simulink model "FDL_Trajectary_Tracking_SBR"  (R2021a)
settings: Solver=VariableStepAuto  StartTime=0.0  StopTime=50  FixedStep=0.01  RelTol=1e-6
values from neighbouring files (symbols this model uses):
  A_v = linear_SBR6voltage_A(I_W_a,I_y,R_m,g,k_e,k_m,l,m_B,m_W,r)    [lqr_control_3DOF.m]
  B_v = linear_SBR6voltage_B(I_W_a,I_W_d,I_y,I_z,R_m,d,k_m,l,m_B,m_W,r)    [lqr_control_3DOF.m]
  C = eye(6)    [lqr_control_3DOF.m]
  C_L = 0    [lqr_control_3DOF.m]
  d = 0.23    [lqr_control_3DOF.m]
  D = zeros(6,2)    [lqr_control_3DOF.m]
  g = 9.81    [lqr_control_3DOF.m]
  I_W_a = 0.0000365    (= 3.65e-05)    [lqr_control_3DOF.m]
  I_W_d = 0.00001825    (= 1.825e-05)    [lqr_control_3DOF.m]
  I_x = 0.007402    [lqr_control_3DOF.m]
  I_y = 0.00429462    [lqr_control_3DOF.m]
  I_z = 0.003350    (= 0.00335)    [lqr_control_3DOF.m]
  k_e = 0.63    [lqr_control_3DOF.m]
  k_m = 0.63    [lqr_control_3DOF.m]
  K_v = lqr(A_v,B_v,Q,R)    [lqr_control_3DOF.m]
  l = 0.045    [lqr_control_3DOF.m]
  m_B = 1.15    [lqr_control_3DOF.m]
  m_W = 0.053    [lqr_control_3DOF.m]
  r = 0.0425    [lqr_control_3DOF.m]
  R_m = 1.25    [lqr_control_3DOF.m]
libraries: aerolibutil x6, vrlib x1
settings Model: SimulationMode=accelerator  Creator=om  LastModifiedBy=jitt7
settings SolverCC: ConcurrentTasks=on  PositivePriorityOrder=on
settings DataIOCC: ReturnWorkspaceOutputs=off
settings OptimizationCC: BlockReduction=off  OptimizeBlockIOStorage=off
settings DebuggingCC: AlgebraicLoopMsg=none  ArtificialAlgebraicLoopMsg=none  SFMachineParentedDataDiag=warning  ArithmeticOperatorsInVariantConditions=warning
settings HardwareCC: ProdBitPerLong=64  ProdLongLongMode=on  ProdHWDeviceType=Intel->x86-64 (Linux 64)
settings SFSimCC: SimUseLocalCustomCode=off  CustomCodeUndefinedFunction=UseInterfaceOnly
settings RTWCC: Description=Simulink Real-Time  SystemTargetFile=slrealtime.tlc  TemplateMakefile=slrealtime_default_tmf  RTWUseLocalCustomCode=off  Toolchain=Simulink Real-Time Toolchain  BuildConfiguration=Faster Runs  CodeExecutionProfiling=on  TargetLang=C++

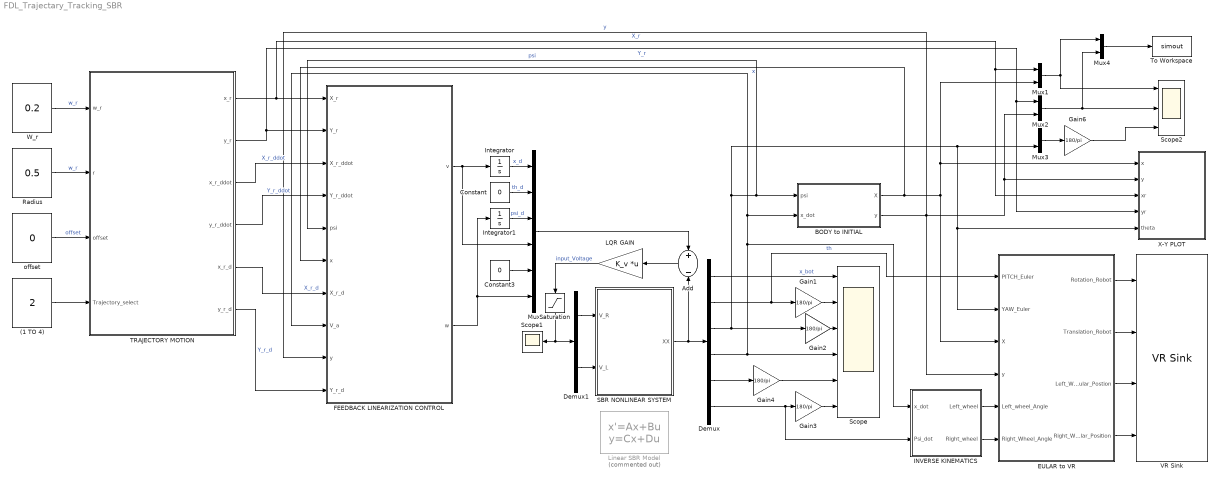
== system FDL_Trajectary_Tracking_SBR ==
  (1 TO 4) : Constant  Value=2
  Add : Sum  Inputs=+-
  BODY to INITIAL : Subsystem
  Constant : Constant  Value=0
  Constant3 : Constant  Value=0
  Demux : Demux  Outputs=6
  Demux1 : Demux  Outputs=2
  EULAR to VR : Subsystem
  FEEDBACK LINEARIZATION CONTROL : Subsystem
  Gain{1..4,6} (5 alike) : Gain  Gain=180/pi
  INVERSE KINEMATICS : Subsystem
  Integrator : Integrator
  Integrator1 : Integrator
  LQR GAIN : Gain  Gain=K_v  Multiplication=Matrix(K*u)
  Linear SBR Model : StateSpace  Commented=on  A=A_v  B=B_v  C=C  D=D  InitialCondition="[0  0  0  0 0 0]"
  Mux : Mux  Inputs=6
  Mux{1..4} (4 alike) : Mux  Inputs=2
  Radius : Constant  Value=0.5
  SBR NONLINEAR SYSTEM : Subsystem
  Saturation : Saturate  UpperLimit=12  LowerLimit=-12
  Scope : Scope  NumInputPorts=6
  Scope1 : Scope
  Scope2 : Scope  NumInputPorts=3
  TRAJECTORY MOTION : Subsystem
  To Workspace : ToWorkspace  VariableName=simout  SampleTime=-1
  VR Sink : vrlib/VR Sink  InstantiateOnLoad=on  SampleTime=0.05  ViewEnable=on  RemoteChange=off  RemoteView=off  FieldsWritten=__1.rotation.4.1.1.double#__1.translation.3.1.1.double#wheel-3.rotation.4.1.1.double#wheel-4.rotation.4.1.1.double  WorldFileName=JitendersirSBR.wrl  AutoView=off  VideoDimensions=[]  AllowVariableSize=off
  W_r : Constant  Value=0.2
  X-Y PLOT : MATLAB Function  TreatAsAtomicUnit=on
  offset : Constant  Value=0
  wires:
  Demux/6 -> INVERSE KINEMATICS/2(Psi_dot), Gain3/1
  Add/1 -> LQR GAIN/1
  Constant/1 -> Mux/2  "th_d"
  Demux/4 -> Scope/4, BODY to INITIAL/2(x_dot), FEEDBACK LINEARIZATION CONTROL/8(V_a), INVERSE KINEMATICS/1(x_dot)
  LQR GAIN/1 -> Saturation/1  "input_Voltage"
  Constant3/1 -> Mux/5
  Demux/2 -> EULAR to VR/1(PITCH_Euler), Gain1/1  "th"
  Demux/1 -> Scope/1  "x_bot"
  Mux/1 -> Add/1
  Gain4/1 -> Scope/5
  Demux/5 -> Gain4/1
  Gain1/1 -> Scope/2
  Gain2/1 -> Scope/3
  Integrator/1 -> Mux/1  "x_d"
  EULAR to VR/2(Translation_Robot) -> VR Sink/2
  EULAR to VR/4(Right_Wheel_Angular_Position) -> VR Sink/4
  EULAR to VR/3(Left_Wheel_Angular_Postion) -> VR Sink/3
  EULAR to VR/1(Rotation_Robot) -> VR Sink/1
  Mux1/1 -> Scope2/1, Mux4/1
  Mux2/1 -> Scope2/2, Mux4/2
  Mux3/1 -> Gain6/1
  Gain6/1 -> Scope2/3
  Demux1/1 -> SBR NONLINEAR SYSTEM/1(V_R)
  Demux1/2 -> SBR NONLINEAR SYSTEM/2(V_L)
  SBR NONLINEAR SYSTEM/1(XX) -> Demux/1, Add/2
  INVERSE KINEMATICS/1(Left_wheel) -> EULAR to VR/5(Left_wheel_Angle)
  INVERSE KINEMATICS/2(Right_wheel) -> EULAR to VR/6(Right_Wheel_Angle)
  BODY to INITIAL/1(X) -> FEEDBACK LINEARIZATION CONTROL/6(x), Mux1/2, X-Y PLOT/1(x), EULAR to VR/3(X)  "x"
  Mux4/1 -> To Workspace/1
  Saturation/1 -> Scope1/1, Demux1/1
  W_r/1 -> TRAJECTORY MOTION/1(w_r)  "w_r"
  TRAJECTORY MOTION/1(x_r) -> Mux1/1, X-Y PLOT/3(xr), FEEDBACK LINEARIZATION CONTROL/1(X_r)  "X_r"
  TRAJECTORY MOTION/2(y_r) -> Mux2/1, X-Y PLOT/4(yr), FEEDBACK LINEARIZATION CONTROL/2(Y_r)  "Y_r"
  BODY to INITIAL/2(y) -> FEEDBACK LINEARIZATION CONTROL/9(y), X-Y PLOT/2(y), Mux2/2, EULAR to VR/4(y)  "y"
  FEEDBACK LINEARIZATION CONTROL/1(v) -> Integrator/1, Mux/4
  FEEDBACK LINEARIZATION CONTROL/2(w) -> Integrator1/1, Mux/6
  TRAJECTORY MOTION/3(x_r_ddot) -> FEEDBACK LINEARIZATION CONTROL/3(X_r_ddot)  "X_r_ddot"
  TRAJECTORY MOTION/4(y_r_ddot) -> FEEDBACK LINEARIZATION CONTROL/4(Y_r_ddot)  "Y_r_ddot"
  TRAJECTORY MOTION/5(x_r_d) -> FEEDBACK LINEARIZATION CONTROL/7(X_r_d)  "X_r_d"
  TRAJECTORY MOTION/6(y_r_d) -> FEEDBACK LINEARIZATION CONTROL/10(Y_r_d)  "Y_r_d"
  offset/1 -> TRAJECTORY MOTION/3(offset)  "offset"
  Radius/1 -> TRAJECTORY MOTION/2(r)  "w_r"
  Demux/3 -> Gain2/1, BODY to INITIAL/1(psi), FEEDBACK LINEARIZATION CONTROL/5(psi), Mux3/2, EULAR to VR/2(YAW_Euler), X-Y PLOT/5(theta)  "psi"
  Integrator1/1 -> Mux/3  "psi_d"
  (1 TO 4)/1 -> TRAJECTORY MOTION/4(Trajectory_select)
  Gain3/1 -> Scope/6

== system FDL_Trajectary_Tracking_SBR/BODY to INITIAL ==
  psi : Inport
  x_dot : Inport  Port=2
  Cos : Trigonometry  Operator=cos
  Integrator : Integrator
  Integrator1 : Integrator
  Multiply : Product
  Multiply1 : Product
  Sin : Trigonometry
  X : Outport  VectorParamsAs1DForOutWhenUnconnected=off
  y : Outport  Port=2  VectorParamsAs1DForOutWhenUnconnected=off
  wires:
  Sin/1 -> Multiply1/1
  Cos/1 -> Multiply/1
  Multiply/1 -> Integrator/1  "X_dot"
  Integrator/1 -> X/1  "X"
  Integrator1/1 -> y/1  "y"
  x_dot/1 -> Multiply/2, Multiply1/2
  psi/1 -> Sin/1, Cos/1
  Multiply1/1 -> Integrator1/1  "Y_ot"

== system FDL_Trajectary_Tracking_SBR/EULAR to VR ==
  PITCH_Euler : Inport
  YAW_Euler : Inport  Port=2
  X : Inport  Port=3
  y : Inport  Port=4
  Left_wheel_Angle : Inport  Port=5
  Right_Wheel_Angle : Inport  Port=6
  EULAR ANGLE : Subsystem
  LEFT WHEEL ROTATION : Subsystem
  RIGHT WHEEL ROTATION : Subsystem
  TRANSLATION : Subsystem
  Rotation_Robot : Outport  VectorParamsAs1DForOutWhenUnconnected=off
  Translation_Robot : Outport  Port=2  VectorParamsAs1DForOutWhenUnconnected=off
  Left_Wheel_Angular_Postion : Outport  Port=3  VectorParamsAs1DForOutWhenUnconnected=off
  Right_Wheel_Angular_Position : Outport  Port=4  VectorParamsAs1DForOutWhenUnconnected=off
  wires:
  PITCH_Euler/1 -> EULAR ANGLE/1(Pitch)  "Pitch"
  YAW_Euler/1 -> EULAR ANGLE/2(Yaw)  "Yaw"
  EULAR ANGLE/1(Rotation_Robot) -> Rotation_Robot/1
  X/1 -> TRANSLATION/1(X)  "X"
  y/1 -> TRANSLATION/2(y)  "y"
  TRANSLATION/1(Translation_Robot) -> Translation_Robot/1
  Left_wheel_Angle/1 -> LEFT WHEEL ROTATION/1(Left_wheel_angle)  "Left_wheel_Angle"
  LEFT WHEEL ROTATION/1(Left_Wheel_Angular_Postion) -> Left_Wheel_Angular_Postion/1
  Right_Wheel_Angle/1 -> RIGHT WHEEL ROTATION/1(Right_Wheel_angle)  "Right_Wheel_angle"
  RIGHT WHEEL ROTATION/1(Right_Wheel_Angular_Position) -> Right_Wheel_Angular_Position/1

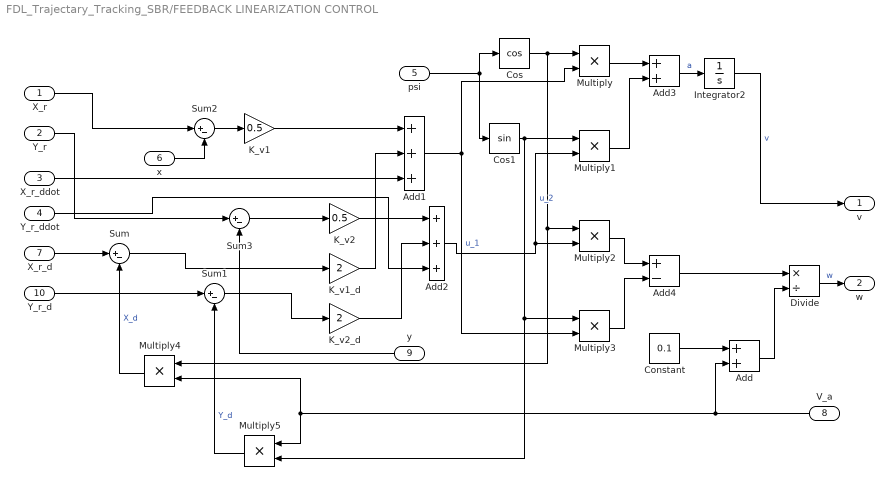
== system FDL_Trajectary_Tracking_SBR/FEEDBACK LINEARIZATION CONTROL ==
  X_r : Inport
  Y_r : Inport  Port=2
  X_r_ddot : Inport  Port=3
  Y_r_ddot : Inport  Port=4
  psi : Inport  Port=5
  x : Inport  Port=6
  X_r_d : Inport  Port=7
  V_a : Inport  Port=8
  y : Inport  Port=9
  Y_r_d : Inport  Port=10
  Add : Sum
  Add1 : Sum  Inputs=+++
  Add2 : Sum  Inputs=+++
  Add3 : Sum
  Add4 : Sum  Inputs=+-
  Constant : Constant  Value=0.1
  Cos : Trigonometry  Operator=cos
  Cos1 : Trigonometry
  Divide : Product  Inputs=*/
  Integrator2 : Integrator
  K_v1 : Gain  Gain=0.5
  K_v1_d : Gain  Gain=2
  K_v2 : Gain  Gain=0.5
  K_v2_d : Gain  Gain=2
  Multiply{,1..5} (6 alike) : Product
  Sum{,1..3} (4 alike) : Sum  Inputs=|+-
  v : Outport
  w : Outport  Port=2
  wires:
  Sum1/1 -> K_v2_d/1
  Integrator2/1 -> v/1  "v"
  Sum/1 -> K_v1_d/1
  Add1/1 -> Multiply/2, Multiply3/2  "u_1"
  psi/1 -> Cos/1, Cos1/1
  Multiply/1 -> Add3/1
  Cos/1 -> Multiply/1, Multiply4/1, Multiply2/1
  Sum2/1 -> K_v1/1
  Sum3/1 -> K_v2/1
  Add2/1 -> Multiply2/2, Multiply1/2  "u_2"
  Multiply1/1 -> Add3/2
  K_v2_d/1 -> Add2/2
  Divide/1 -> w/1  "w"
  Multiply2/1 -> Add4/1
  K_v1/1 -> Add1/1
  Cos1/1 -> Multiply5/2, Multiply3/1, Multiply1/1
  K_v2/1 -> Add2/1
  Multiply3/1 -> Add4/2
  K_v1_d/1 -> Add1/2
  Y_r_d/1 -> Sum1/1
  Add4/1 -> Divide/1
  V_a/1 -> Add/2, Multiply4/2, Multiply5/1
  Y_r/1 -> Sum3/1
  Multiply4/1 -> Sum/2  "X_d"
  Multiply5/1 -> Sum1/2  "Y_d"
  X_r/1 -> Sum2/1
  y/1 -> Sum3/2
  Add3/1 -> Integrator2/1  "a"
  X_r_ddot/1 -> Add1/3
  Y_r_ddot/1 -> Add2/3
  X_r_d/1 -> Sum/1
  x/1 -> Sum2/2
  Add/1 -> Divide/2
  Constant/1 -> Add/1

== system FDL_Trajectary_Tracking_SBR/INVERSE KINEMATICS ==
  x_dot : Inport
  Psi_dot : Inport  Port=2
  Add1 : Sum
  Add2 : Sum  Inputs=+-
  Gain3 : Gain  Gain=1/r
  Gain5 : Gain  Gain=d/(2*r)
  Integrator : Integrator
  Integrator1 : Integrator
  Left_wheel : Outport  VectorParamsAs1DForOutWhenUnconnected=off
  Right_wheel : Outport  Port=2  VectorParamsAs1DForOutWhenUnconnected=off
  wires:
  Gain3/1 -> Add1/1, Add2/1
  Integrator1/1 -> Right_wheel/1
  Psi_dot/1 -> Gain5/1
  Add1/1 -> Integrator1/1
  Gain5/1 -> Add2/2, Add1/2
  Add2/1 -> Integrator/1
  x_dot/1 -> Gain3/1
  Integrator/1 -> Left_wheel/1

== system FDL_Trajectary_Tracking_SBR/SBR NONLINEAR SYSTEM ==
  V_R : Inport
  V_L : Inport  Port=2
  Mux : Mux  Inputs=6
  Psi_DD 3rd EOM : Subsystem
  Voltage to Torque : Subsystem
  X_DD 1st EOM : Subsystem
  th_DD 2st EOM : Subsystem
  XX : Outport  VectorParamsAs1DForOutWhenUnconnected=off
  wires:
  Psi_DD 3rd EOM/1(Psi_dot) -> X_DD 1st EOM/6(Psi_dot), th_DD 2st EOM/5(Psi_dot), Mux/6  "Psi_dot_p"
  X_DD 1st EOM/2(X_dot) -> Voltage to Torque/2(X_dot_p), Mux/4, Psi_DD 3rd EOM/1(X_dot), th_DD 2st EOM/4(X_dot)  "X_dot_p"
  th_DD 2st EOM/1(theta) -> Mux/2, Psi_DD 3rd EOM/3(theta), X_DD 1st EOM/3(theta)  "theta_p"
  th_DD 2st EOM/3(theta_dot) -> Mux/5, Psi_DD 3rd EOM/5(theta_dot), X_DD 1st EOM/5(theta_dot)  "theta_dot_p"
  th_DD 2st EOM/2(theta_ddot) -> X_DD 1st EOM/4(theta_ddot)
  X_DD 1st EOM/3(X_dd) -> th_DD 2st EOM/3(X_dd)
  X_DD 1st EOM/1(XX) -> Mux/1  "X_p"
  Voltage to Torque/2(T_L) -> Psi_DD 3rd EOM/4(T_L), X_DD 1st EOM/2(T_L), th_DD 2st EOM/2(T_L)
  Voltage to Torque/1(T_R) -> Psi_DD 3rd EOM/2(T_R), th_DD 2st EOM/1(T_R), X_DD 1st EOM/1(T_R)
  V_R/1 -> Voltage to Torque/1(V_R)  "V_R"
  V_L/1 -> Voltage to Torque/3(V_L)  "V_L"
  Mux/1 -> XX/1
  Psi_DD 3rd EOM/2(Psi) -> Mux/3

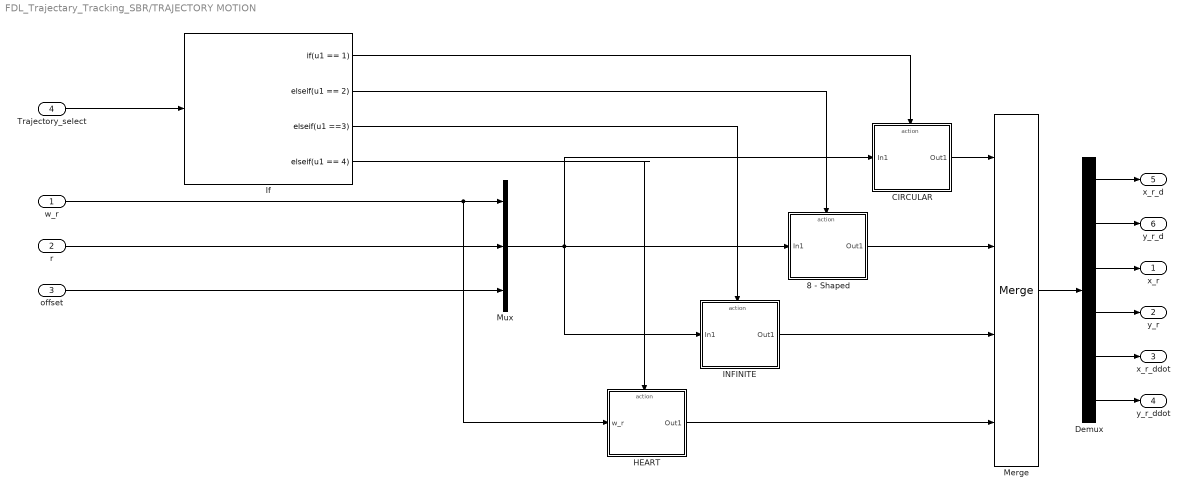
== system FDL_Trajectary_Tracking_SBR/TRAJECTORY MOTION ==
  w_r : Inport
  r : Inport  Port=2
  offset : Inport  Port=3
  Trajectory_select : Inport  Port=4
  8 - Shaped : Subsystem  TreatAsAtomicUnit=on
  CIRCULAR : Subsystem  TreatAsAtomicUnit=on
  Demux : Demux  Outputs=6
  HEART : Subsystem  TreatAsAtomicUnit=on
  INFINITE : Subsystem  TreatAsAtomicUnit=on
  If : If  IfExpression=u1 == 1  ElseIfExpressions=u1 == 2, u1 ==3, u1 == 4  ShowElse=off
  Merge : Merge  Inputs=4
  Mux : Mux  Inputs=3
  x_r : Outport  VectorParamsAs1DForOutWhenUnconnected=off
  y_r : Outport  Port=2  VectorParamsAs1DForOutWhenUnconnected=off
  x_r_ddot : Outport  Port=3  VectorParamsAs1DForOutWhenUnconnected=off
  y_r_ddot : Outport  Port=4  VectorParamsAs1DForOutWhenUnconnected=off
  x_r_d : Outport  Port=5  VectorParamsAs1DForOutWhenUnconnected=off
  y_r_d : Outport  Port=6  VectorParamsAs1DForOutWhenUnconnected=off
  wires:
  Demux/1 -> x_r_d/1
  Demux/2 -> y_r_d/1
  Demux/3 -> x_r/1
  Demux/4 -> y_r/1
  Demux/5 -> x_r_ddot/1
  Demux/6 -> y_r_ddot/1
  Merge/1 -> Demux/1
  CIRCULAR/1(Out1) -> Merge/1
  r/1 -> Mux/2
  w_r/1 -> HEART/1(w_r), Mux/1
  offset/1 -> Mux/3
  Mux/1 -> INFINITE/1(In1), 8 - Shaped/1(In1), CIRCULAR/1(In1)
  8 - Shaped/1(Out1) -> Merge/2
  INFINITE/1(Out1) -> Merge/3
  If/1 -> CIRCULAR/Action
  If/2 -> 8 - Shaped/Action
  If/3 -> INFINITE/Action
  Trajectory_select/1 -> If/1
  HEART/1(Out1) -> Merge/4
  If/4 -> HEART/Action

== system FDL_Trajectary_Tracking_SBR/EULAR to VR/EULAR ANGLE ==
  Pitch : Inport
  Yaw : Inport  Port=2
  Constant : Constant  Value=90
  Euler to VR : Subsystem
  Gain : Gain  Gain=pi/180
  Gain1 : Gain  Gain=-1
  Gain2 : Gain  Gain=-1
  Mux : Mux  Inputs=3
  Rate Transition : RateTransition
  Rotation_Robot : Outport  VectorParamsAs1DForOutWhenUnconnected=off
  wires:
  Constant/1 -> Gain/1  "Roll_90"
  Gain2/1 -> Mux/3
  Gain1/1 -> Mux/2
  Gain/1 -> Mux/1
  Mux/1 -> Euler to VR/1(Euler Angles)
  Rate Transition/1 -> Rotation_Robot/1  "Rotation_Robot"
  Euler to VR/1(Axis Angle) -> Rate Transition/1
  Pitch/1 -> Gain1/1
  Yaw/1 -> Gain2/1

== system FDL_Trajectary_Tracking_SBR/EULAR to VR/LEFT WHEEL ROTATION ==
  Left_wheel_angle : Inport
  Constant6 : Constant  Value=-90
  Constant7 : Constant  Value=0
  Euler to VR1 : Subsystem
  Gain3 : Gain  Gain=pi/180
  Gain4 : Gain  Gain=-pi/180
  Gain5 : Gain
  Mux2 : Mux  Inputs=3
  Rate Transition2 : RateTransition
  Left_Wheel_Angular_Postion : Outport  VectorParamsAs1DForOutWhenUnconnected=off
  wires:
  Left_wheel_angle/1 -> Gain5/1
  Euler to VR1/1(Axis Angle) -> Rate Transition2/1
  Gain5/1 -> Mux2/3
  Mux2/1 -> Euler to VR1/1(Euler Angles)  "Left_Wheel"
  Gain4/1 -> Mux2/2
  Constant6/1 -> Gain3/1  "-90"
  Gain3/1 -> Mux2/1
  Rate Transition2/1 -> Left_Wheel_Angular_Postion/1  "Left_Wheel_Angular_Postion"
  Constant7/1 -> Gain4/1  "0"

== system FDL_Trajectary_Tracking_SBR/EULAR to VR/RIGHT WHEEL ROTATION ==
  Right_Wheel_angle : Inport
  Constant1 : Constant  Value=0
  Constant9 : Constant  Value=90
  Euler to VR2 : Subsystem
  Gain6 : Gain  Gain=pi/180
  Gain7 : Gain  Gain=-pi/180
  Gain8 : Gain
  Mux3 : Mux  Inputs=3
  Rate Transition3 : RateTransition
  Right_Wheel_Angular_Position : Outport  VectorParamsAs1DForOutWhenUnconnected=off
  wires:
  Gain7/1 -> Mux3/2
  Constant1/1 -> Gain7/1
  Gain8/1 -> Mux3/3
  Euler to VR2/1(Axis Angle) -> Rate Transition3/1
  Right_Wheel_angle/1 -> Gain8/1
  Gain6/1 -> Mux3/1
  Rate Transition3/1 -> Right_Wheel_Angular_Position/1  "Right_Wheel_Angular_Position"
  Mux3/1 -> Euler to VR2/1(Euler Angles)  "Right Wheel"
  Constant9/1 -> Gain6/1  "90"

== system FDL_Trajectary_Tracking_SBR/EULAR to VR/TRANSLATION ==
  X : Inport
  y : Inport  Port=2
  Axes to VR Axes : Subsystem
  Constant5 : Constant  Value=0
  Gain10 : Gain  Gain=7
  Gain9 : Gain  Gain=-7
  Mux1 : Mux  Inputs=3
  Rate Transition1 : RateTransition
  Translation_Robot : Outport  VectorParamsAs1DForOutWhenUnconnected=off
  wires:
  Axes to VR Axes/1(Xe VR) -> Rate Transition1/1
  Mux1/1 -> Axes to VR Axes/1(Xe)
  Gain10/1 -> Mux1/1
  Rate Transition1/1 -> Translation_Robot/1  "Translation_Robot"
  Gain9/1 -> Mux1/2
  X/1 -> Gain10/1
  y/1 -> Gain9/1
  Constant5/1 -> Mux1/3  "z"

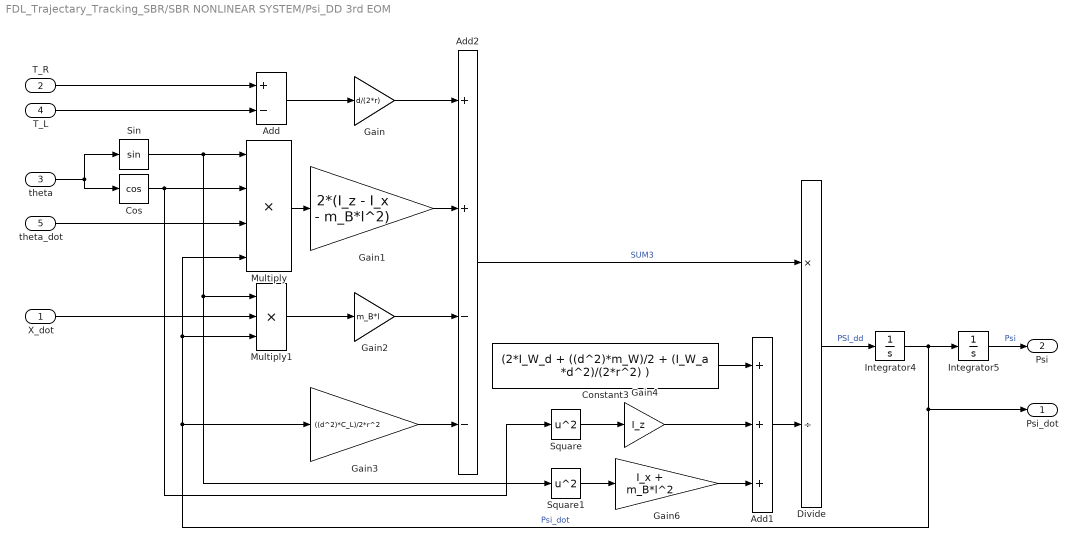
== system FDL_Trajectary_Tracking_SBR/SBR NONLINEAR SYSTEM/Psi_DD 3rd EOM ==
  X_dot : Inport
  T_R : Inport  Port=2
  theta : Inport  Port=3
  T_L : Inport  Port=4
  theta_dot : Inport  Port=5
  Add : Sum  Inputs=+-
  Add1 : Sum  Inputs=+++
  Add2 : Sum  Inputs=++--
  Constant3 : Constant  Value=(2*I_W_d + ((d^2)*m_W)/2 + (I_W_a *d^2)/(2*r^2) )
  Cos : Trigonometry  Operator=cos
  Divide : Product  Inputs=*/
  Gain : Gain  Gain=d/(2*r)
  Gain1 : Gain  Gain=2*(I_z - I_x - m_B*l^2)
  Gain2 : Gain  Gain=m_B*l
  Gain3 : Gain  Gain=((d^2)*C_L)/2*r^2
  Gain4 : Gain  Gain=I_z
  Gain6 : Gain  Gain=I_x + m_B*l^2
  Integrator4 : Integrator
  Integrator5 : Integrator
  Multiply : Product  Inputs=4
  Multiply1 : Product  Inputs=3
  Sin : Trigonometry
  Square : Math  Operator=square  SignedPower=on  SaturateOnIntegerOverflow=on
  Square1 : Math  Operator=square  SignedPower=on  SaturateOnIntegerOverflow=on
  Psi_dot : Outport  VectorParamsAs1DForOutWhenUnconnected=off
  Psi : Outport  Port=2  VectorParamsAs1DForOutWhenUnconnected=off
  wires:
  theta/1 -> Cos/1, Sin/1
  Constant3/1 -> Add1/1
  Multiply/1 -> Gain1/1
  Cos/1 -> Square/1, Multiply/2
  Multiply1/1 -> Gain2/1
  Gain2/1 -> Add2/3
  Add2/1 -> Divide/1  "SUM3"
  Integrator5/1 -> Psi/1  "Psi"
  T_R/1 -> Add/1
  Sin/1 -> Square1/1, Multiply1/1, Multiply/1
  Integrator4/1 -> Psi_dot/1, Gain3/1, Multiply1/3, Multiply/4, Integrator5/1  "Psi_dot"
  Gain3/1 -> Add2/4
  Gain/1 -> Add2/1
  Divide/1 -> Integrator4/1  "PSI_dd"
  Add/1 -> Gain/1
  X_dot/1 -> Multiply1/2
  theta_dot/1 -> Multiply/3
  Gain1/1 -> Add2/2
  Square/1 -> Gain4/1
  T_L/1 -> Add/2
  Square1/1 -> Gain6/1
  Add1/1 -> Divide/2
  Gain6/1 -> Add1/3
  Gain4/1 -> Add1/2

== system FDL_Trajectary_Tracking_SBR/SBR NONLINEAR SYSTEM/Voltage to Torque ==
  V_R : Inport
  X_dot_p : Inport  Port=2
  V_L : Inport  Port=3
  Add : Sum  Inputs=+-
  Add1 : Sum  Inputs=+-
  Gain : Gain  Gain=k_m/R_m
  Gain1 : Gain  Gain=(k_m*k_e)/(r*R_m)
  Gain2 : Gain  Gain=k_m/R_m
  Gain3 : Gain  Gain=(k_m*k_e)/(r*R_m)
  T_R : Outport  VectorParamsAs1DForOutWhenUnconnected=off
  T_L : Outport  Port=2  VectorParamsAs1DForOutWhenUnconnected=off
  wires:
  X_dot_p/1 -> Gain3/1, Gain1/1
  Gain/1 -> Add/1
  Add/1 -> T_R/1  "T_R"
  Gain2/1 -> Add1/1
  V_R/1 -> Gain/1
  Gain3/1 -> Add1/2
  Gain1/1 -> Add/2
  V_L/1 -> Gain2/1
  Add1/1 -> T_L/1  "T_L"

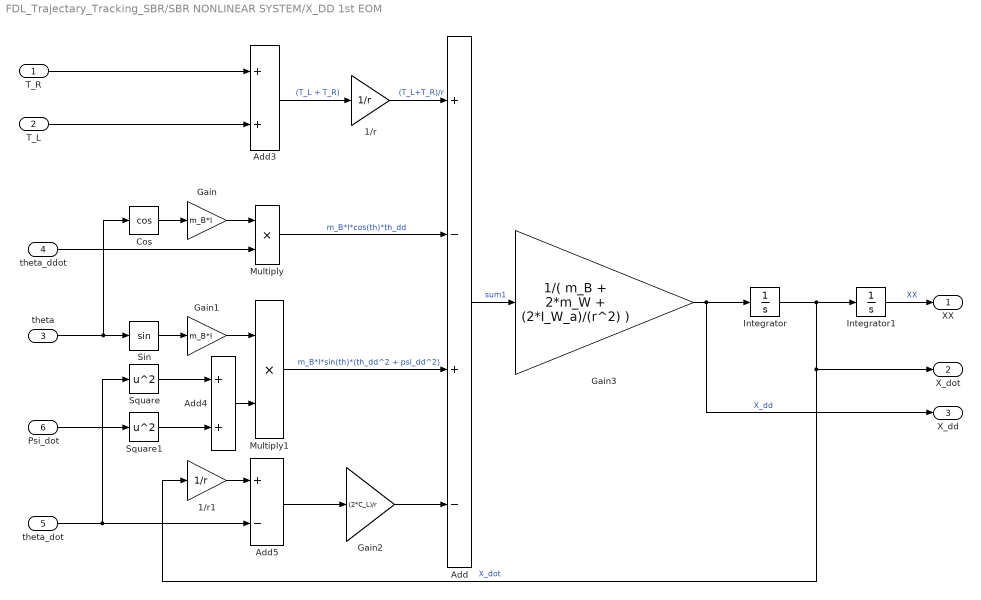
== system FDL_Trajectary_Tracking_SBR/SBR NONLINEAR SYSTEM/X_DD 1st EOM ==
  T_R : Inport
  T_L : Inport  Port=2
  theta : Inport  Port=3
  theta_ddot : Inport  Port=4
  theta_dot : Inport  Port=5
  Psi_dot : Inport  Port=6
  1/r : Gain  Gain=1/r
  1/r1 : Gain  Gain=1/r
  Add : Sum  Inputs=+-+-
  Add3 : Sum
  Add4 : Sum
  Add5 : Sum  Inputs=+-
  Cos : Trigonometry  Operator=cos
  Gain : Gain  Gain=m_B*l
  Gain1 : Gain  Gain=m_B*l
  Gain2 : Gain  Gain=(2*C_L)/r
  Gain3 : Gain  Gain="1/( m_B + 2*m_W + (2*I_W_a)/(r^2)  )"
  Integrator : Integrator
  Integrator1 : Integrator
  Multiply : Product
  Multiply1 : Product
  Sin : Trigonometry
  Square : Math  Operator=square  SignedPower=on  SaturateOnIntegerOverflow=on
  Square1 : Math  Operator=square  SignedPower=on  SaturateOnIntegerOverflow=on
  XX : Outport  VectorParamsAs1DForOutWhenUnconnected=off
  X_dot : Outport  Port=2  VectorParamsAs1DForOutWhenUnconnected=off
  X_dd : Outport  Port=3  VectorParamsAs1DForOutWhenUnconnected=off
  wires:
  Add4/1 -> Multiply1/2
  Gain1/1 -> Multiply1/1
  Multiply1/1 -> Add/3  "m_B*l*sin(th)*(th_dd^2 + psi_dd^2)"
  Gain3/1 -> X_dd/1, Integrator/1  "X_dd"
  Add3/1 -> 1/r/1  "(T_L + T_R)"
  Integrator/1 -> 1/r1/1, X_dot/1, Integrator1/1  "X_dot"
  Sin/1 -> Gain1/1
  theta/1 -> Sin/1, Cos/1
  Square1/1 -> Add4/2
  1/r1/1 -> Add5/1
  Add5/1 -> Gain2/1
  Square/1 -> Add4/1
  Multiply/1 -> Add/2  "m_B*l*cos(th)*th_dd"
  Add/1 -> Gain3/1  "sum1"
  Gain/1 -> Multiply/1
  theta_dot/1 -> Square/1, Add5/2
  1/r/1 -> Add/1  "(T_L+T_R)/r"
  Cos/1 -> Gain/1
  Gain2/1 -> Add/4
  Psi_dot/1 -> Square1/1
  T_L/1 -> Add3/2
  theta_ddot/1 -> Multiply/2
  Integrator1/1 -> XX/1  "XX"
  T_R/1 -> Add3/1

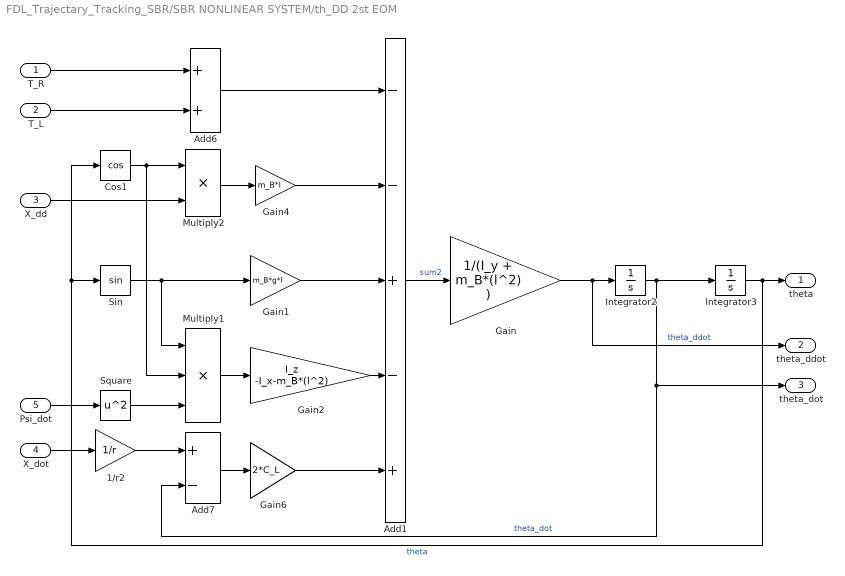
== system FDL_Trajectary_Tracking_SBR/SBR NONLINEAR SYSTEM/th_DD 2st EOM ==
  T_R : Inport
  T_L : Inport  Port=2
  X_dd : Inport  Port=3
  X_dot : Inport  Port=4
  Psi_dot : Inport  Port=5
  1/r2 : Gain  Gain=1/r
  Add1 : Sum  Inputs=--+-+
  Add6 : Sum
  Add7 : Sum  Inputs=+-
  Cos1 : Trigonometry  Operator=cos
  Gain : Gain  Gain=1/(I_y + m_B*(l^2) )
  Gain1 : Gain  Gain=m_B*g*l
  Gain2 : Gain  Gain=I_z -I_x-m_B*(l^2)
  Gain4 : Gain  Gain=m_B*l
  Gain6 : Gain  Gain=2*C_L
  Integrator2 : Integrator
  Integrator3 : Integrator
  Multiply1 : Product  Inputs=3
  Multiply2 : Product
  Sin : Trigonometry
  Square : Math  Operator=square  SignedPower=on  SaturateOnIntegerOverflow=on
  theta : Outport  VectorParamsAs1DForOutWhenUnconnected=off
  theta_ddot : Outport  Port=2  VectorParamsAs1DForOutWhenUnconnected=off
  theta_dot : Outport  Port=3  VectorParamsAs1DForOutWhenUnconnected=off
  wires:
  Cos1/1 -> Multiply1/2, Multiply2/1
  Gain4/1 -> Add1/2
  Sin/1 -> Multiply1/1, Gain1/1
  1/r2/1 -> Add7/1
  Gain/1 -> theta_ddot/1, Integrator2/1  "theta_ddot"
  Integrator3/1 -> Cos1/1, Sin/1, theta/1  "theta"
  Integrator2/1 -> Integrator3/1, theta_dot/1, Add7/2  "theta_dot"
  Add7/1 -> Gain6/1
  Gain6/1 -> Add1/5
  Multiply2/1 -> Gain4/1
  Square/1 -> Multiply1/3
  Add6/1 -> Add1/1
  Add1/1 -> Gain/1  "sum2"
  Psi_dot/1 -> Square/1
  Multiply1/1 -> Gain2/1
  Gain1/1 -> Add1/3
  X_dd/1 -> Multiply2/2
  T_L/1 -> Add6/2
  T_R/1 -> Add6/1
  X_dot/1 -> 1/r2/1
  Gain2/1 -> Add1/4

== system FDL_Trajectary_Tracking_SBR/TRAJECTORY MOTION/8 - Shaped ==
  In1 : Inport
  Action Port : ActionPort  ActionPortLabel=elseif(u1 == 2)
  8 - Shaped TRAJECTORY : Subsystem
  Demux : Demux  Outputs=3
  Mux : Mux  Inputs=6
  Out1 : Outport
  wires:
  8 - Shaped TRAJECTORY/1(x_r_d) -> Mux/1
  8 - Shaped TRAJECTORY/2(y_r_d) -> Mux/2
  8 - Shaped TRAJECTORY/3(x_r) -> Mux/3
  8 - Shaped TRAJECTORY/4(y_r) -> Mux/4
  8 - Shaped TRAJECTORY/5(x_r_ddot) -> Mux/5
  8 - Shaped TRAJECTORY/6(y_r_ddot) -> Mux/6
  Mux/1 -> Out1/1
  Demux/1 -> 8 - Shaped TRAJECTORY/1(W_r)
  Demux/2 -> 8 - Shaped TRAJECTORY/2(Radius)
  Demux/3 -> 8 - Shaped TRAJECTORY/3(offset)
  In1/1 -> Demux/1

== system FDL_Trajectary_Tracking_SBR/TRAJECTORY MOTION/CIRCULAR ==
  In1 : Inport
  Action Port : ActionPort  ActionPortLabel=if(u1 == 1)
  CIRCULAR TRAJECTORY : Subsystem
  Demux : Demux  Outputs=3
  Mux : Mux  Inputs=6
  Out1 : Outport
  wires:
  CIRCULAR TRAJECTORY/1(x_r_d) -> Mux/1
  CIRCULAR TRAJECTORY/2(y_r_d) -> Mux/2
  CIRCULAR TRAJECTORY/3(x_r) -> Mux/3
  CIRCULAR TRAJECTORY/4(y_r) -> Mux/4
  CIRCULAR TRAJECTORY/5(x_r_ddot) -> Mux/5
  CIRCULAR TRAJECTORY/6(y_r_ddot) -> Mux/6
  Mux/1 -> Out1/1
  Demux/1 -> CIRCULAR TRAJECTORY/1(W_r)
  Demux/2 -> CIRCULAR TRAJECTORY/2(r)
  Demux/3 -> CIRCULAR TRAJECTORY/3(offset)
  In1/1 -> Demux/1

== system FDL_Trajectary_Tracking_SBR/TRAJECTORY MOTION/HEART ==
  w_r : Inport
  Action Port : ActionPort  ActionPortLabel=elseif( u1 == 4)
  Integrator : Integrator
  MATLAB Function : MATLAB Function  TreatAsAtomicUnit=on
  Mux : Mux  Inputs=6
  Out1 : Outport
  wires:
  MATLAB Function/1(x_r_d) -> Mux/1
  MATLAB Function/2(y_r_d) -> Mux/2
  MATLAB Function/3(x_r) -> Mux/3
  MATLAB Function/4(y_r) -> Mux/4
  MATLAB Function/5(x_r_ddot) -> Mux/5
  MATLAB Function/6(y_r_ddot) -> Mux/6
  Mux/1 -> Out1/1
  w_r/1 -> Integrator/1, MATLAB Function/1(w)
  Integrator/1 -> MATLAB Function/2(theta)

== system FDL_Trajectary_Tracking_SBR/TRAJECTORY MOTION/INFINITE ==
  In1 : Inport
  Action Port : ActionPort  ActionPortLabel=elseif( u1 ==3)
  Demux : Demux  Outputs=3
  INFINITE - Shaped TRAJECTORY : Subsystem
  Mux : Mux  Inputs=6
  Out1 : Outport
  wires:
  INFINITE - Shaped TRAJECTORY/1(x_r_d) -> Mux/1
  INFINITE - Shaped TRAJECTORY/2(y_r_d) -> Mux/2
  INFINITE - Shaped TRAJECTORY/3(x_r) -> Mux/3
  INFINITE - Shaped TRAJECTORY/4(y_r) -> Mux/4
  INFINITE - Shaped TRAJECTORY/5(x_r_ddot) -> Mux/5
  INFINITE - Shaped TRAJECTORY/6(y_r_ddot) -> Mux/6
  Mux/1 -> Out1/1
  Demux/1 -> INFINITE - Shaped TRAJECTORY/1(W_r)
  Demux/2 -> INFINITE - Shaped TRAJECTORY/2(Radius)
  Demux/3 -> INFINITE - Shaped TRAJECTORY/3(offset)
  In1/1 -> Demux/1

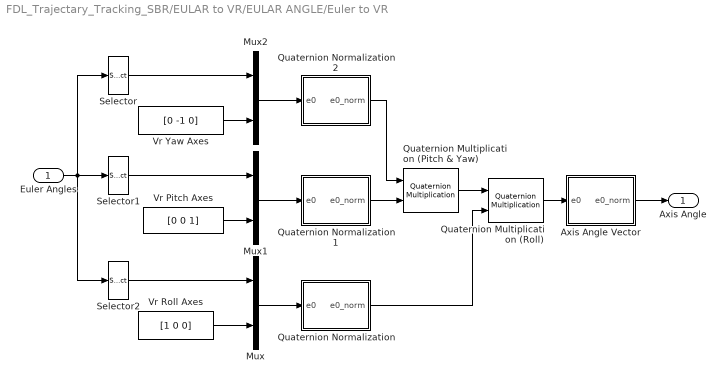
== system FDL_Trajectary_Tracking_SBR/EULAR to VR/EULAR ANGLE/Euler to VR ==
  Euler Angles : Inport
  Axis Angle Vector : Subsystem
  Mux : Mux  Inputs=2
  Mux1 : Mux  Inputs=2
  Mux2 : Mux  Inputs=2
  Quaternion Multiplication (Pitch & Yaw) : aerolibutil/Quaternion Multiplication
  Quaternion Multiplication (Roll) : aerolibutil/Quaternion Multiplication
  Quaternion Normalization : Subsystem
  Quaternion Normalization1 : Subsystem
  Quaternion Normalization2 : Subsystem
  Selector : Selector  InputPortWidth=3  IndexOptions=Index vector (dialog)  Indices=[3]  OutputSizes=1
  Selector1 : Selector  InputPortWidth=3  IndexOptions=Index vector (dialog)  Indices=[2]  OutputSizes=1
  Selector2 : Selector  InputPortWidth=3  IndexOptions=Index vector (dialog)  Indices=[1]  OutputSizes=1
  Vr Pitch Axes : Constant  Value=[0 0 1]
  Vr Roll Axes : Constant  Value=[1 0 0]
  Vr Yaw Axes : Constant  Value=[0 -1 0]
  Axis Angle : Outport  VectorParamsAs1DForOutWhenUnconnected=off
  wires:
  Quaternion Multiplication (Roll)/1 -> Axis Angle Vector/1(e0)
  Axis Angle Vector/1(e0_norm) -> Axis Angle/1
  Quaternion Normalization/1(e0_norm) -> Quaternion Multiplication (Roll)/2
  Quaternion Normalization2/1(e0_norm) -> Quaternion Multiplication (Pitch & Yaw)/1
  Quaternion Normalization1/1(e0_norm) -> Quaternion Multiplication (Pitch & Yaw)/2
  Mux2/1 -> Quaternion Normalization2/1(e0)
  Mux1/1 -> Quaternion Normalization1/1(e0)
  Mux/1 -> Quaternion Normalization/1(e0)
  Selector/1 -> Mux2/1
  Vr Yaw Axes/1 -> Mux2/2
  Selector1/1 -> Mux1/1
  Vr Pitch Axes/1 -> Mux1/2
  Selector2/1 -> Mux/1
  Vr Roll Axes/1 -> Mux/2
  Euler Angles/1 -> Selector2/1, Selector1/1, Selector/1
  Quaternion Multiplication (Pitch & Yaw)/1 -> Quaternion Multiplication (Roll)/1

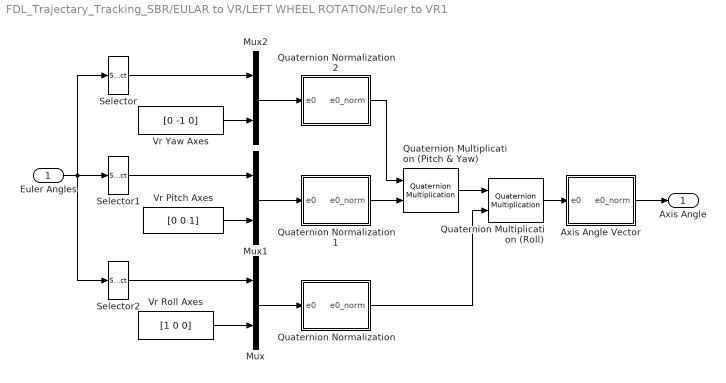
== system FDL_Trajectary_Tracking_SBR/EULAR to VR/LEFT WHEEL ROTATION/Euler to VR1 ==
  Euler Angles : Inport
  Axis Angle Vector : Subsystem
  Mux : Mux  Inputs=2
  Mux1 : Mux  Inputs=2
  Mux2 : Mux  Inputs=2
  Quaternion Multiplication (Pitch & Yaw) : aerolibutil/Quaternion Multiplication
  Quaternion Multiplication (Roll) : aerolibutil/Quaternion Multiplication
  Quaternion Normalization : Subsystem
  Quaternion Normalization1 : Subsystem
  Quaternion Normalization2 : Subsystem
  Selector : Selector  InputPortWidth=3  IndexOptions=Index vector (dialog)  Indices=[3]  OutputSizes=1
  Selector1 : Selector  InputPortWidth=3  IndexOptions=Index vector (dialog)  Indices=[2]  OutputSizes=1
  Selector2 : Selector  InputPortWidth=3  IndexOptions=Index vector (dialog)  Indices=[1]  OutputSizes=1
  Vr Pitch Axes : Constant  Value=[0 0 1]
  Vr Roll Axes : Constant  Value=[1 0 0]
  Vr Yaw Axes : Constant  Value=[0 -1 0]
  Axis Angle : Outport  VectorParamsAs1DForOutWhenUnconnected=off
  wires:
  Quaternion Multiplication (Roll)/1 -> Axis Angle Vector/1(e0)
  Axis Angle Vector/1(e0_norm) -> Axis Angle/1
  Quaternion Normalization/1(e0_norm) -> Quaternion Multiplication (Roll)/2
  Quaternion Normalization2/1(e0_norm) -> Quaternion Multiplication (Pitch & Yaw)/1
  Quaternion Normalization1/1(e0_norm) -> Quaternion Multiplication (Pitch & Yaw)/2
  Mux2/1 -> Quaternion Normalization2/1(e0)
  Mux1/1 -> Quaternion Normalization1/1(e0)
  Mux/1 -> Quaternion Normalization/1(e0)
  Selector/1 -> Mux2/1
  Vr Yaw Axes/1 -> Mux2/2
  Selector1/1 -> Mux1/1
  Vr Pitch Axes/1 -> Mux1/2
  Selector2/1 -> Mux/1
  Vr Roll Axes/1 -> Mux/2
  Euler Angles/1 -> Selector2/1, Selector1/1, Selector/1
  Quaternion Multiplication (Pitch & Yaw)/1 -> Quaternion Multiplication (Roll)/1

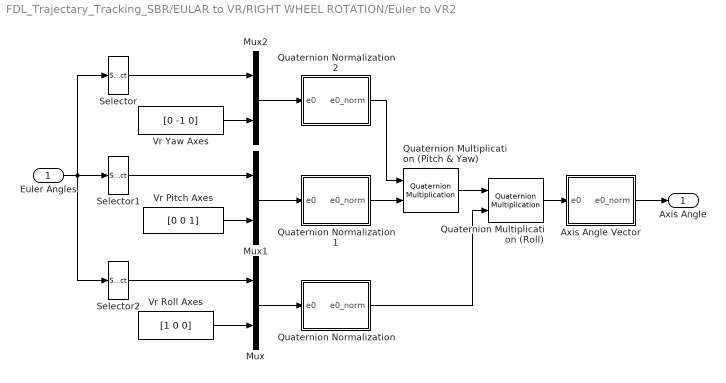
== system FDL_Trajectary_Tracking_SBR/EULAR to VR/RIGHT WHEEL ROTATION/Euler to VR2 ==
  Euler Angles : Inport
  Axis Angle Vector : Subsystem
  Mux : Mux  Inputs=2
  Mux1 : Mux  Inputs=2
  Mux2 : Mux  Inputs=2
  Quaternion Multiplication (Pitch & Yaw) : aerolibutil/Quaternion Multiplication
  Quaternion Multiplication (Roll) : aerolibutil/Quaternion Multiplication
  Quaternion Normalization : Subsystem
  Quaternion Normalization1 : Subsystem
  Quaternion Normalization2 : Subsystem
  Selector : Selector  InputPortWidth=3  IndexOptions=Index vector (dialog)  Indices=[3]  OutputSizes=1
  Selector1 : Selector  InputPortWidth=3  IndexOptions=Index vector (dialog)  Indices=[2]  OutputSizes=1
  Selector2 : Selector  InputPortWidth=3  IndexOptions=Index vector (dialog)  Indices=[1]  OutputSizes=1
  Vr Pitch Axes : Constant  Value=[0 0 1]
  Vr Roll Axes : Constant  Value=[1 0 0]
  Vr Yaw Axes : Constant  Value=[0 -1 0]
  Axis Angle : Outport  VectorParamsAs1DForOutWhenUnconnected=off
  wires:
  Quaternion Multiplication (Roll)/1 -> Axis Angle Vector/1(e0)
  Axis Angle Vector/1(e0_norm) -> Axis Angle/1
  Quaternion Normalization/1(e0_norm) -> Quaternion Multiplication (Roll)/2
  Quaternion Normalization2/1(e0_norm) -> Quaternion Multiplication (Pitch & Yaw)/1
  Quaternion Normalization1/1(e0_norm) -> Quaternion Multiplication (Pitch & Yaw)/2
  Mux2/1 -> Quaternion Normalization2/1(e0)
  Mux1/1 -> Quaternion Normalization1/1(e0)
  Mux/1 -> Quaternion Normalization/1(e0)
  Selector/1 -> Mux2/1
  Vr Yaw Axes/1 -> Mux2/2
  Selector1/1 -> Mux1/1
  Vr Pitch Axes/1 -> Mux1/2
  Selector2/1 -> Mux/1
  Vr Roll Axes/1 -> Mux/2
  Euler Angles/1 -> Selector2/1, Selector1/1, Selector/1
  Quaternion Multiplication (Pitch & Yaw)/1 -> Quaternion Multiplication (Roll)/1

== system FDL_Trajectary_Tracking_SBR/EULAR to VR/TRANSLATION/Axes to VR Axes ==
  Xe : Inport
  Demux : Demux  Outputs=3
      settings: DisplayOption=none
  Mux : Mux  Inputs=3
  rad-->deg1 : Gain  Gain=-1  SaturateOnIntegerOverflow=on  OutDataTypeStr=Inherit: Same as input  ParamDataTypeStr=Inherit: Same as input
  Xe VR : Outport  VectorParamsAs1DForOutWhenUnconnected=off
  wires:
  Xe/1 -> Demux/1
  Demux/1 -> Mux/1
  Demux/3 -> rad-->deg1/1
  Mux/1 -> Xe VR/1
  rad-->deg1/1 -> Mux/2
  Demux/2 -> Mux/3

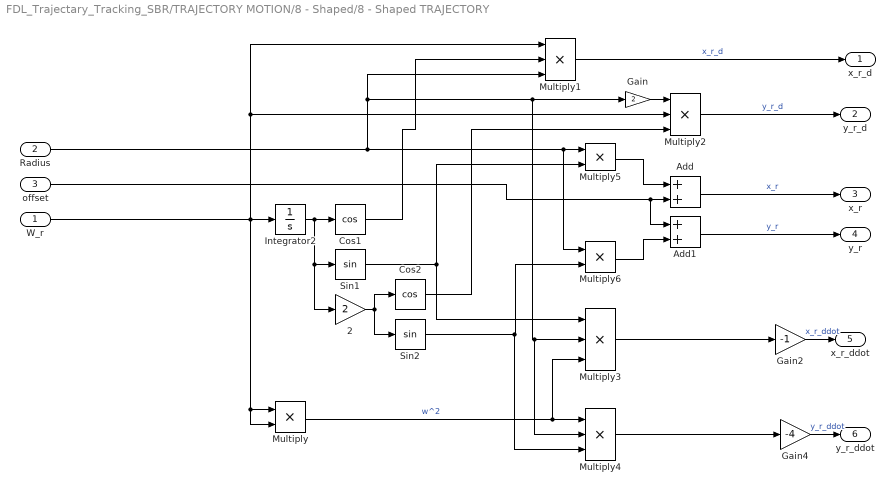
== system FDL_Trajectary_Tracking_SBR/TRAJECTORY MOTION/8 - Shaped/8 - Shaped TRAJECTORY ==
  W_r : Inport
  Radius : Inport  Port=2
  offset : Inport  Port=3
  2 : Gain  Gain=2
  Add : Sum
  Add1 : Sum
  Cos1 : Trigonometry  Operator=cos
  Cos2 : Trigonometry  Operator=cos
  Gain : Gain  Gain=2
  Gain2 : Gain  Gain=-1
  Gain4 : Gain  Gain=-4
  Integrator2 : Integrator
  Multiply : Product
  Multiply{1..4} (4 alike) : Product  Inputs=3
  Multiply5 : Product
  Multiply6 : Product
  Sin1 : Trigonometry
  Sin2 : Trigonometry
  x_r_d : Outport
  y_r_d : Outport  Port=2
  x_r : Outport  Port=3
  y_r : Outport  Port=4
  x_r_ddot : Outport  Port=5
  y_r_ddot : Outport  Port=6
  wires:
  Multiply3/1 -> Gain2/1
  Integrator2/1 -> Cos1/1, 2/1, Sin1/1
  Sin1/1 -> Multiply5/2, Multiply3/1
  Multiply/1 -> Multiply3/3, Multiply4/1  "w^2"
  Multiply4/1 -> Gain4/1
  Add/1 -> x_r/1  "x_r"
  Multiply2/1 -> y_r_d/1  "y_r_d"
  Gain4/1 -> y_r_ddot/1  "y_r_ddot"
  Gain2/1 -> x_r_ddot/1  "x_r_ddot"
  Multiply1/1 -> x_r_d/1  "x_r_d"
  Add1/1 -> y_r/1  "y_r"
  2/1 -> Sin2/1, Cos2/1
  Multiply5/1 -> Add/1
  Multiply6/1 -> Add1/2
  Sin2/1 -> Multiply4/3, Multiply6/2
  Radius/1 -> Multiply1/3, Multiply4/2, Multiply3/2, Gain/1, Multiply6/1, Multiply5/1
  offset/1 -> Add1/1, Add/2
  Gain/1 -> Multiply2/1
  W_r/1 -> Multiply/2, Multiply/1, Integrator2/1, Multiply2/2, Multiply1/1
  Cos1/1 -> Multiply1/2
  Cos2/1 -> Multiply2/3

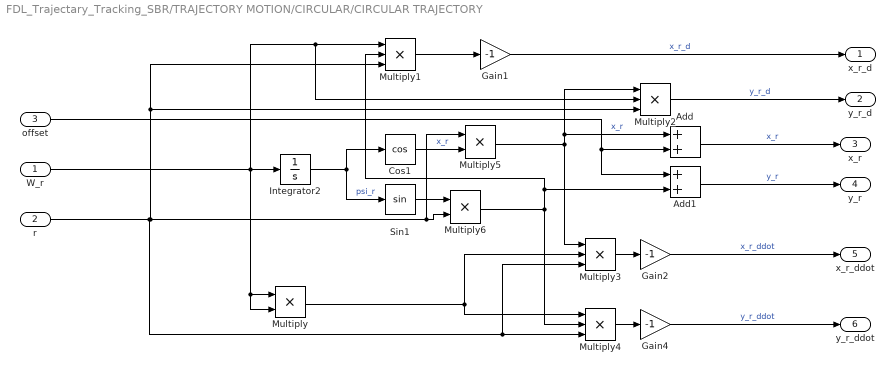
== system FDL_Trajectary_Tracking_SBR/TRAJECTORY MOTION/CIRCULAR/CIRCULAR TRAJECTORY ==
  W_r : Inport
  r : Inport  Port=2
  offset : Inport  Port=3
  Add : Sum
  Add1 : Sum
  Cos1 : Trigonometry  Operator=cos
  Gain1 : Gain  Gain=-1
  Gain2 : Gain  Gain=-1
  Gain4 : Gain  Gain=-1
  Integrator2 : Integrator
  Multiply : Product
  Multiply{1..4} (4 alike) : Product  Inputs=3
  Multiply5 : Product
  Multiply6 : Product
  Sin1 : Trigonometry
  x_r_d : Outport
  y_r_d : Outport  Port=2
  x_r : Outport  Port=3
  y_r : Outport  Port=4
  x_r_ddot : Outport  Port=5
  y_r_ddot : Outport  Port=6
  wires:
  Multiply6/1 -> Multiply1/2, Add1/2, Multiply4/2
  Multiply3/1 -> Gain2/1
  Integrator2/1 -> Sin1/1, Cos1/1  "psi_r"
  W_r/1 -> Multiply/2, Multiply/1, Integrator2/1, Multiply2/2, Multiply1/1
  Multiply5/1 -> Multiply3/1, Add/1, Multiply2/1  "x_r"
  Multiply/1 -> Multiply3/2, Multiply4/1
  Multiply1/1 -> Gain1/1
  Multiply4/1 -> Gain4/1
  Add/1 -> x_r/1  "x_r"
  Multiply2/1 -> y_r_d/1  "y_r_d"
  Gain4/1 -> y_r_ddot/1  "y_r_ddot"
  Gain2/1 -> x_r_ddot/1  "x_r_ddot"
  Gain1/1 -> x_r_d/1  "x_r_d"
  Add1/1 -> y_r/1  "y_r"
  offset/1 -> Add1/1, Add/2
  r/1 -> Multiply3/3, Multiply4/3, Multiply5/1, Multiply6/2, Multiply1/3, Multiply2/3
  Cos1/1 -> Multiply5/2  "x_r"
  Sin1/1 -> Multiply6/1

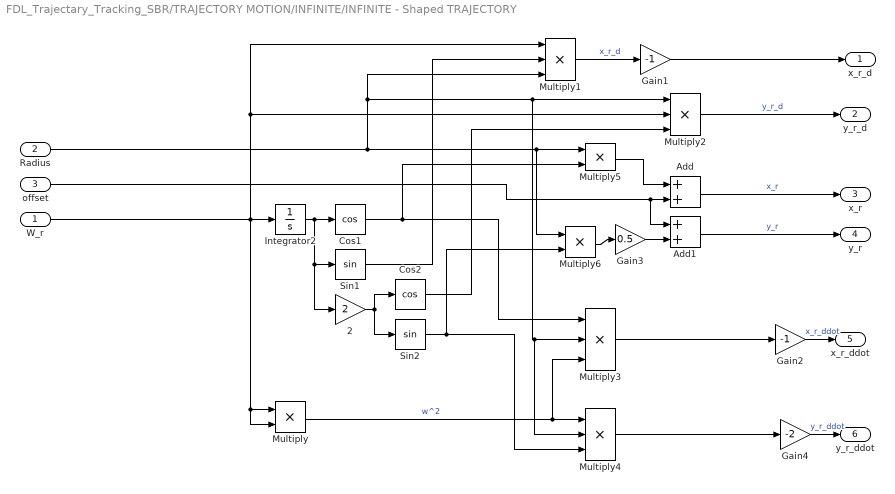
== system FDL_Trajectary_Tracking_SBR/TRAJECTORY MOTION/INFINITE/INFINITE - Shaped TRAJECTORY ==
  W_r : Inport
  Radius : Inport  Port=2
  offset : Inport  Port=3
  2 : Gain  Gain=2
  Add : Sum
  Add1 : Sum
  Cos1 : Trigonometry  Operator=cos
  Cos2 : Trigonometry  Operator=cos
  Gain1 : Gain  Gain=-1
  Gain2 : Gain  Gain=-1
  Gain3 : Gain  Gain=0.5
  Gain4 : Gain  Gain=-2
  Integrator2 : Integrator
  Multiply : Product
  Multiply{1..4} (4 alike) : Product  Inputs=3
  Multiply5 : Product
  Multiply6 : Product
  Sin1 : Trigonometry
  Sin2 : Trigonometry
  x_r_d : Outport
  y_r_d : Outport  Port=2
  x_r : Outport  Port=3
  y_r : Outport  Port=4
  x_r_ddot : Outport  Port=5
  y_r_ddot : Outport  Port=6
  wires:
  Multiply3/1 -> Gain2/1
  Integrator2/1 -> Cos1/1, 2/1, Sin1/1
  Sin1/1 -> Multiply1/2
  Multiply/1 -> Multiply3/3, Multiply4/1  "w^2"
  Multiply4/1 -> Gain4/1
  Add/1 -> x_r/1  "x_r"
  Multiply2/1 -> y_r_d/1  "y_r_d"
  Gain4/1 -> y_r_ddot/1  "y_r_ddot"
  Gain2/1 -> x_r_ddot/1  "x_r_ddot"
  Multiply1/1 -> Gain1/1  "x_r_d"
  Add1/1 -> y_r/1  "y_r"
  2/1 -> Sin2/1, Cos2/1
  Multiply5/1 -> Add/1
  Sin2/1 -> Multiply6/2, Multiply4/3
  offset/1 -> Add1/1, Add/2
  Radius/1 -> Multiply1/3, Multiply2/1, Multiply4/2, Multiply3/2, Multiply5/1, Multiply6/1
  W_r/1 -> Multiply/2, Multiply/1, Integrator2/1, Multiply2/2, Multiply1/1
  Cos1/1 -> Multiply3/1, Multiply5/2
  Cos2/1 -> Multiply2/3
  Gain1/1 -> x_r_d/1
  Multiply6/1 -> Gain3/1
  Gain3/1 -> Add1/2

== system FDL_Trajectary_Tracking_SBR/EULAR to VR/EULAR ANGLE/Euler to VR/Axis Angle Vector ==
  e0 : Inport
  2 : Gain  Gain=2  SaturateOnIntegerOverflow=on  OutDataTypeStr=Inherit: Same as input  ParamDataTypeStr=Inherit: Same as input
  Constant : Constant  Value=1e-6
  Demux : Demux  Outputs=[1 3 ]
      settings: DisplayOption=none
  Mux : Mux  Inputs=2
  Product : Product  Inputs=*/  InputSameDT=on  SaturateOnIntegerOverflow=on  OutDataTypeStr=Inherit: Same as first input
  Switch : Switch  Criteria=u2 ~= 0
  Trigonometric Function : Trigonometry
  Trigonometric Function2 : Trigonometry  Operator=acos
  e0_norm : Outport  VectorParamsAs1DForOutWhenUnconnected=off
  wires:
  Demux/1 -> Trigonometric Function2/1
  Demux/2 -> Product/1
  Mux/1 -> e0_norm/1
  Product/1 -> Mux/1
  2/1 -> Mux/2
  Trigonometric Function/1 -> Switch/1, Switch/2
  Trigonometric Function2/1 -> Trigonometric Function/1, 2/1
  e0/1 -> Demux/1
  Constant/1 -> Switch/3
  Switch/1 -> Product/2

== system FDL_Trajectary_Tracking_SBR/EULAR to VR/EULAR ANGLE/Euler to VR/Quaternion Normalization ==
  e0 : Inport
  1/2 : Gain  Gain=1/2  SaturateOnIntegerOverflow=on  OutDataTypeStr=Inherit: Same as input  ParamDataTypeStr=Inherit: Same as input
  Demux : Demux  Outputs=[1 3]
      settings: DisplayOption=none
  Mux : Mux  Inputs=2
  Product : Product  InputSameDT=on  SaturateOnIntegerOverflow=on  OutDataTypeStr=Inherit: Same as first input
  Trigonometric Function : Trigonometry
  Trigonometric Function1 : Trigonometry  Operator=cos
  e0_norm : Outport  VectorParamsAs1DForOutWhenUnconnected=off
  wires:
  Trigonometric Function1/1 -> Mux/1
  Demux/2 -> Product/2
  Demux/1 -> 1/2/1
  Mux/1 -> e0_norm/1
  Product/1 -> Mux/2
  Trigonometric Function/1 -> Product/1
  1/2/1 -> Trigonometric Function1/1, Trigonometric Function/1
  e0/1 -> Demux/1

== system FDL_Trajectary_Tracking_SBR/EULAR to VR/EULAR ANGLE/Euler to VR/Quaternion Normalization1 ==
  e0 : Inport
  1/2 : Gain  Gain=1/2  SaturateOnIntegerOverflow=on  OutDataTypeStr=Inherit: Same as input  ParamDataTypeStr=Inherit: Same as input
  Demux : Demux  Outputs=[1 3]
      settings: DisplayOption=none
  Mux : Mux  Inputs=2
  Product : Product  InputSameDT=on  SaturateOnIntegerOverflow=on  OutDataTypeStr=Inherit: Same as first input
  Trigonometric Function : Trigonometry
  Trigonometric Function1 : Trigonometry  Operator=cos
  e0_norm : Outport  VectorParamsAs1DForOutWhenUnconnected=off
  wires:
  e0/1 -> Demux/1
  1/2/1 -> Trigonometric Function/1, Trigonometric Function1/1
  Trigonometric Function/1 -> Product/1
  Product/1 -> Mux/2
  Mux/1 -> e0_norm/1
  Demux/1 -> 1/2/1
  Demux/2 -> Product/2
  Trigonometric Function1/1 -> Mux/1

== system FDL_Trajectary_Tracking_SBR/EULAR to VR/EULAR ANGLE/Euler to VR/Quaternion Normalization2 ==
  e0 : Inport
  1/2 : Gain  Gain=1/2  SaturateOnIntegerOverflow=on  OutDataTypeStr=Inherit: Same as input  ParamDataTypeStr=Inherit: Same as input
  Demux : Demux  Outputs=[1 3]
      settings: DisplayOption=none
  Mux : Mux  Inputs=2
  Product : Product  InputSameDT=on  SaturateOnIntegerOverflow=on  OutDataTypeStr=Inherit: Same as first input
  Trigonometric Function : Trigonometry
  Trigonometric Function1 : Trigonometry  Operator=cos
  e0_norm : Outport  VectorParamsAs1DForOutWhenUnconnected=off
  wires:
  Trigonometric Function1/1 -> Mux/1
  Demux/2 -> Product/2
  Demux/1 -> 1/2/1
  Mux/1 -> e0_norm/1
  Product/1 -> Mux/2
  Trigonometric Function/1 -> Product/1
  1/2/1 -> Trigonometric Function1/1, Trigonometric Function/1
  e0/1 -> Demux/1

== system FDL_Trajectary_Tracking_SBR/EULAR to VR/LEFT WHEEL ROTATION/Euler to VR1/Axis Angle Vector ==
  e0 : Inport
  2 : Gain  Gain=2  SaturateOnIntegerOverflow=on  OutDataTypeStr=Inherit: Same as input  ParamDataTypeStr=Inherit: Same as input
  Constant : Constant  Value=1e-6
  Demux : Demux  Outputs=[1 3 ]
      settings: DisplayOption=none
  Mux : Mux  Inputs=2
  Product : Product  Inputs=*/  InputSameDT=on  SaturateOnIntegerOverflow=on  OutDataTypeStr=Inherit: Same as first input
  Switch : Switch  Criteria=u2 ~= 0
  Trigonometric Function : Trigonometry
  Trigonometric Function2 : Trigonometry  Operator=acos
  e0_norm : Outport  VectorParamsAs1DForOutWhenUnconnected=off
  wires:
  Demux/1 -> Trigonometric Function2/1
  Demux/2 -> Product/1
  Mux/1 -> e0_norm/1
  Product/1 -> Mux/1
  2/1 -> Mux/2
  Trigonometric Function/1 -> Switch/1, Switch/2
  Trigonometric Function2/1 -> Trigonometric Function/1, 2/1
  e0/1 -> Demux/1
  Constant/1 -> Switch/3
  Switch/1 -> Product/2

== system FDL_Trajectary_Tracking_SBR/EULAR to VR/LEFT WHEEL ROTATION/Euler to VR1/Quaternion Normalization ==
  e0 : Inport
  1/2 : Gain  Gain=1/2  SaturateOnIntegerOverflow=on  OutDataTypeStr=Inherit: Same as input  ParamDataTypeStr=Inherit: Same as input
  Demux : Demux  Outputs=[1 3]
      settings: DisplayOption=none
  Mux : Mux  Inputs=2
  Product : Product  InputSameDT=on  SaturateOnIntegerOverflow=on  OutDataTypeStr=Inherit: Same as first input
  Trigonometric Function : Trigonometry
  Trigonometric Function1 : Trigonometry  Operator=cos
  e0_norm : Outport  VectorParamsAs1DForOutWhenUnconnected=off
  wires:
  Trigonometric Function1/1 -> Mux/1
  Demux/2 -> Product/2
  Demux/1 -> 1/2/1
  Mux/1 -> e0_norm/1
  Product/1 -> Mux/2
  Trigonometric Function/1 -> Product/1
  1/2/1 -> Trigonometric Function1/1, Trigonometric Function/1
  e0/1 -> Demux/1

== system FDL_Trajectary_Tracking_SBR/EULAR to VR/LEFT WHEEL ROTATION/Euler to VR1/Quaternion Normalization1 ==
  e0 : Inport
  1/2 : Gain  Gain=1/2  SaturateOnIntegerOverflow=on  OutDataTypeStr=Inherit: Same as input  ParamDataTypeStr=Inherit: Same as input
  Demux : Demux  Outputs=[1 3]
      settings: DisplayOption=none
  Mux : Mux  Inputs=2
  Product : Product  InputSameDT=on  SaturateOnIntegerOverflow=on  OutDataTypeStr=Inherit: Same as first input
  Trigonometric Function : Trigonometry
  Trigonometric Function1 : Trigonometry  Operator=cos
  e0_norm : Outport  VectorParamsAs1DForOutWhenUnconnected=off
  wires:
  e0/1 -> Demux/1
  1/2/1 -> Trigonometric Function/1, Trigonometric Function1/1
  Trigonometric Function/1 -> Product/1
  Product/1 -> Mux/2
  Mux/1 -> e0_norm/1
  Demux/1 -> 1/2/1
  Demux/2 -> Product/2
  Trigonometric Function1/1 -> Mux/1

== system FDL_Trajectary_Tracking_SBR/EULAR to VR/LEFT WHEEL ROTATION/Euler to VR1/Quaternion Normalization2 ==
  e0 : Inport
  1/2 : Gain  Gain=1/2  SaturateOnIntegerOverflow=on  OutDataTypeStr=Inherit: Same as input  ParamDataTypeStr=Inherit: Same as input
  Demux : Demux  Outputs=[1 3]
      settings: DisplayOption=none
  Mux : Mux  Inputs=2
  Product : Product  InputSameDT=on  SaturateOnIntegerOverflow=on  OutDataTypeStr=Inherit: Same as first input
  Trigonometric Function : Trigonometry
  Trigonometric Function1 : Trigonometry  Operator=cos
  e0_norm : Outport  VectorParamsAs1DForOutWhenUnconnected=off
  wires:
  Trigonometric Function1/1 -> Mux/1
  Demux/2 -> Product/2
  Demux/1 -> 1/2/1
  Mux/1 -> e0_norm/1
  Product/1 -> Mux/2
  Trigonometric Function/1 -> Product/1
  1/2/1 -> Trigonometric Function1/1, Trigonometric Function/1
  e0/1 -> Demux/1

== system FDL_Trajectary_Tracking_SBR/EULAR to VR/RIGHT WHEEL ROTATION/Euler to VR2/Axis Angle Vector ==
  e0 : Inport
  2 : Gain  Gain=2  SaturateOnIntegerOverflow=on  OutDataTypeStr=Inherit: Same as input  ParamDataTypeStr=Inherit: Same as input
  Constant : Constant  Value=1e-6
  Demux : Demux  Outputs=[1 3 ]
      settings: DisplayOption=none
  Mux : Mux  Inputs=2
  Product : Product  Inputs=*/  InputSameDT=on  SaturateOnIntegerOverflow=on  OutDataTypeStr=Inherit: Same as first input
  Switch : Switch  Criteria=u2 ~= 0
  Trigonometric Function : Trigonometry
  Trigonometric Function2 : Trigonometry  Operator=acos
  e0_norm : Outport  VectorParamsAs1DForOutWhenUnconnected=off
  wires:
  Demux/1 -> Trigonometric Function2/1
  Demux/2 -> Product/1
  Mux/1 -> e0_norm/1
  Product/1 -> Mux/1
  2/1 -> Mux/2
  Trigonometric Function/1 -> Switch/1, Switch/2
  Trigonometric Function2/1 -> Trigonometric Function/1, 2/1
  e0/1 -> Demux/1
  Constant/1 -> Switch/3
  Switch/1 -> Product/2

== system FDL_Trajectary_Tracking_SBR/EULAR to VR/RIGHT WHEEL ROTATION/Euler to VR2/Quaternion Normalization ==
  e0 : Inport
  1/2 : Gain  Gain=1/2  SaturateOnIntegerOverflow=on  OutDataTypeStr=Inherit: Same as input  ParamDataTypeStr=Inherit: Same as input
  Demux : Demux  Outputs=[1 3]
      settings: DisplayOption=none
  Mux : Mux  Inputs=2
  Product : Product  InputSameDT=on  SaturateOnIntegerOverflow=on  OutDataTypeStr=Inherit: Same as first input
  Trigonometric Function : Trigonometry
  Trigonometric Function1 : Trigonometry  Operator=cos
  e0_norm : Outport  VectorParamsAs1DForOutWhenUnconnected=off
  wires:
  Trigonometric Function1/1 -> Mux/1
  Demux/2 -> Product/2
  Demux/1 -> 1/2/1
  Mux/1 -> e0_norm/1
  Product/1 -> Mux/2
  Trigonometric Function/1 -> Product/1
  1/2/1 -> Trigonometric Function1/1, Trigonometric Function/1
  e0/1 -> Demux/1

== system FDL_Trajectary_Tracking_SBR/EULAR to VR/RIGHT WHEEL ROTATION/Euler to VR2/Quaternion Normalization1 ==
  e0 : Inport
  1/2 : Gain  Gain=1/2  SaturateOnIntegerOverflow=on  OutDataTypeStr=Inherit: Same as input  ParamDataTypeStr=Inherit: Same as input
  Demux : Demux  Outputs=[1 3]
      settings: DisplayOption=none
  Mux : Mux  Inputs=2
  Product : Product  InputSameDT=on  SaturateOnIntegerOverflow=on  OutDataTypeStr=Inherit: Same as first input
  Trigonometric Function : Trigonometry
  Trigonometric Function1 : Trigonometry  Operator=cos
  e0_norm : Outport  VectorParamsAs1DForOutWhenUnconnected=off
  wires:
  e0/1 -> Demux/1
  1/2/1 -> Trigonometric Function/1, Trigonometric Function1/1
  Trigonometric Function/1 -> Product/1
  Product/1 -> Mux/2
  Mux/1 -> e0_norm/1
  Demux/1 -> 1/2/1
  Demux/2 -> Product/2
  Trigonometric Function1/1 -> Mux/1

== system FDL_Trajectary_Tracking_SBR/EULAR to VR/RIGHT WHEEL ROTATION/Euler to VR2/Quaternion Normalization2 ==
  e0 : Inport
  1/2 : Gain  Gain=1/2  SaturateOnIntegerOverflow=on  OutDataTypeStr=Inherit: Same as input  ParamDataTypeStr=Inherit: Same as input
  Demux : Demux  Outputs=[1 3]
      settings: DisplayOption=none
  Mux : Mux  Inputs=2
  Product : Product  InputSameDT=on  SaturateOnIntegerOverflow=on  OutDataTypeStr=Inherit: Same as first input
  Trigonometric Function : Trigonometry
  Trigonometric Function1 : Trigonometry  Operator=cos
  e0_norm : Outport  VectorParamsAs1DForOutWhenUnconnected=off
  wires:
  Trigonometric Function1/1 -> Mux/1
  Demux/2 -> Product/2
  Demux/1 -> 1/2/1
  Mux/1 -> e0_norm/1
  Product/1 -> Mux/2
  Trigonometric Function/1 -> Product/1
  1/2/1 -> Trigonometric Function1/1, Trigonometric Function/1
  e0/1 -> Demux/1

== matlab function FDL_Trajectary_Tracking_SBR/TRAJECTORY MOTION/HEART/MATLAB Function ==
  data: w input; theta input; x_r_d output; y_r_d output; x_r output; y_r output; x_r_ddot output; y_r_ddot output
function [x_r_d,y_r_d,x_r,y_r,x_r_ddot,y_r_ddot] = heart_traj(w,theta)
th = theta;
x_r = (sin(th))^3;
y_r = (13*cos(th)-5*cos(2*th)-2*cos(3*th)-cos(4*th))/16;

x_r_d = 3*w*cos(th)*(sin(th))^2;
y_r_d = (5/8)*w*sin(2*th) - (13/16)*w*sin(th) + (3/8)*w*sin(3*th) + (w/4)*sin(4*th);

x_r_ddot = 6*(w^2)*sin(th)*(cos(th))^2 - 3*(w^2)*(sin(th))^3;
y_r_ddot = (5/4)*(w^2)*cos(2*th)-(13/16)*(w^2)*cos(th)+(9/8)*(w^2)*cos(3*th)+(w^2)*cos(4*th);

== matlab function FDL_Trajectary_Tracking_SBR/X-Y PLOT ==
  settings: updateMethod=DISCRETE
  data: x input; y input; xr input; yr input; theta input
% Code is written by JITENDRA SINGH
% India 
% this code written for making the animation of Mobile Robot model, 
% all units are in meters, in this code of example we are using 'patch'
% function for animate the trajectory of Mobile robot
% {Thanks to MATLAB}
function plotXY(x,y,xr,yr,theta)
persistent xp yp x_r y_r;
if isempty(xp)
    xp =x;
end
if isempty(yp)
    yp =y;
end
if isempty(x_r)
    x_r =xr;
end
if isempty(y_r)
    y_r =yr;
end

th = theta;
W = 0.4; % width of robot
H = 0.3; % Hight of robot
x_r = [x_r xr];
y_r = [y_r yr];
xp = [xp x];
yp = [yp y];
coder.extrinsic('patch'); %Declare patch as extrinsic
Ri = [cos(th) -sin(th) 0;
      sin(th) cos(th)  0;
       0       0       1];     % rotation matrix to rotate the coordinates of base 
base_triangle = [-W/2 W/2 -W/2; % Coordinates of Base 
                 -H/2  0  +H/2;
                   0   0    0];
base_rot = Ri*base_triangle;
base_trans = [x x x;
              y y y;
              0 0 0];  
base = base_trans + base_rot;         
clf
hold on
grid on;
axis square
title('Trajectory Tracking (Jitendra)','FontSize',16)
ylabel('X(m)','FontSize',16);
xlabel('Y(m)','FontSize',16);
xlim([-1.5,1.5]);
ylim([-1.5,1.5])
% Plot robot
p1 = patch([base(1,:)],[base(2,:)],[base(3,:)],'m');
alpha(p1,0.5);
plot(x_r,y_r,'b--','LineWidth',2)
plot(xp,yp,'r','LineWidth',1.3)
%legend('reference','actual')

%drawnow('limitrate')
